simulink model "tank_warmup"  (R2024b)
settings: Solver=ode15s  StartTime=0.0  StopTime=100  RelTol=1e-3
undefined symbols (not defined in the file): AC_tank_weight, Ambient_temp
libraries: fl_lib x11, nesl_utility x7, SimscapeFluids_lib x3
settings Model: Creator=MW  LastModifiedBy=MW

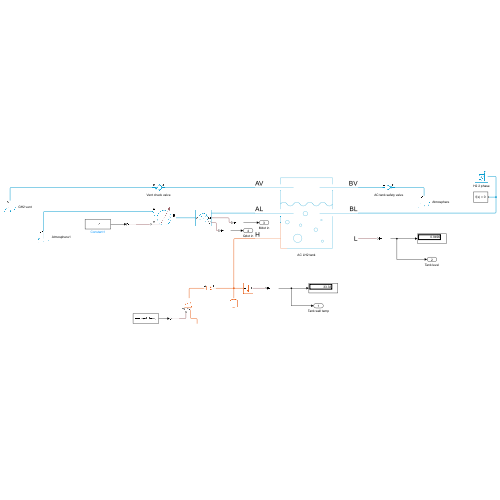
[thumbnail: Simulink's stored preview of the top-level diagram]
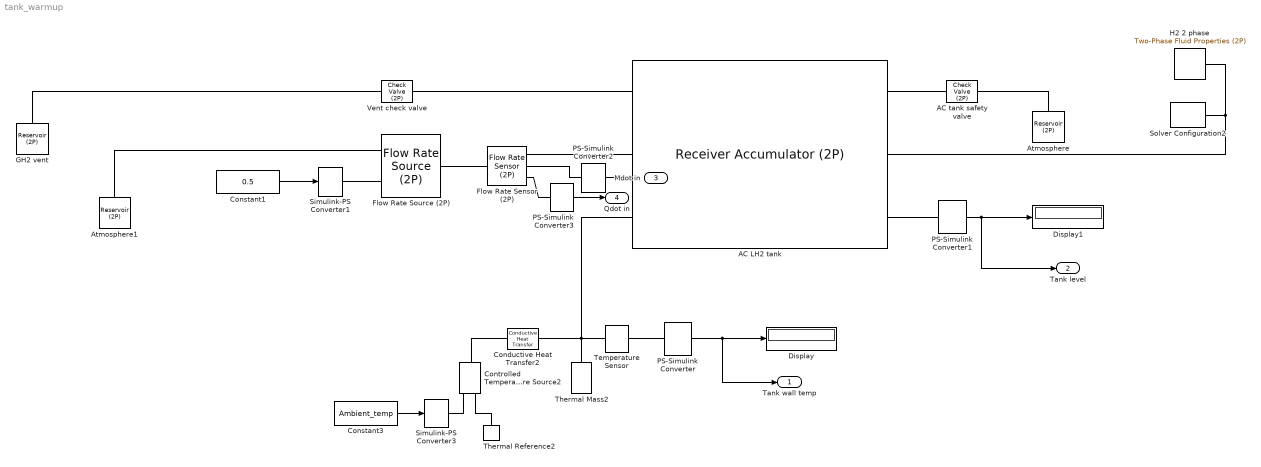
== system tank_warmup ==
  AC LH2 tank : SimscapeFluids_lib/Two-Phase Fluid/Tanks & Accumulators/Receiver Accumulator (2P)  volume=AC_tank_volume m^3  tank_area=AC_tank_cross_sectional_area m^2  area_AV=AC_return_line_port_inner_area m^2  area_BV=return_pipe_inner_area m^2  area_AL=AC_supply_line_port_inner_area m^2  area_BL=AC_engine_feed_port_inner_area m^2  V_frac_liq_error=simscape.enum.assert.action.none  V_frac_liq_min=0.05  V_frac_liq_max=0.95  V_frac_smooth=0.01  p_crit_error=simscape.enum.assert.action.error  hc_vap=AC_tank_vapour_heat_transfer_coeff W/(K*m^2)  hc_liq=AC_tank_liquid_heat_transfer_coeff W/(K*m^2)  p_init=3 bar  fraction_spec=fluids.two_phase_fluid.tanks_accumulators.enum.LiquidFractionSpec.Volume  M_frac_liq_init=0.5  V_frac_liq_init=0.9  saturated_init=false  energy_spec=fluids.two_phase_fluid.tanks_accumulators.enum.EnergySpec.Temperature  delta_T_sub_init=5 deltaK  delta_T_sup_init=5 deltaK  T_liq_init=20 K  T_vap_init=27 K  h_liq_init=400 kJ/kg  h_vap_init=2700 kJ/kg  u_liq_init=400 kJ/kg  u_vap_init=2700 kJ/kg  tau_vap_cond=0.1 s
      settings: InternalSimscapePortConfiguration="{\"Bottom\":[],\"Left\":[{\"id\":\"AV\",\"label\":\"AV\",\"type\":\"foundation.two_phase_fluid.two_phase_fluid\"},{\"id\":\"AL\",\"label\":\"AL\",\"type\":\"foundation.two_phase_fluid.two_phase_fluid\"},{\"id\":\"H\",\"label\":\"H\",\"type\":\"foundation.thermal.thermal\"}],\"Right\":[{\"id\":\"BV\",\"label\":\"BV\",\"type\":\"foundation.two_phase_fluid.two_phase_fluid\"},{\"id\":\"BL\",\"label\":\"BL\",\"type\":\"foundation.two_phase_fluid.two_phase_fluid\"},{\"id\":\"L\",\"label\":\"L\",\"type\":\"output\"}],\"Top\":[]}"
  AC tank safety valve : SimscapeFluids_lib/Two-Phase Fluid/Valves & Orifices/Directional Control Valves/Check Valve (2P)  liquid_valve_parameterization=fluids.two_phase_fluid.valves_orifices.enum.LiquidPressureValveParameterization.LinearArea  opening_pressure_spec=fluids.two_phase_fluid.valves_orifices.enum.PressureControlSpec.PressureDifferential  p_crack_differential=4.5 bar  p_crack_gauge=0.1 MPa  p_max_differential=4.9 bar  p_max_gauge=0.2 MPa  mdot_nominal_max=0.1 kg/s  delta_p_nominal_max=0.001 MPa  valve_area_max=AC_vent_valve_orifice_area m^2  p_diff_TLU=[0.2 : 0.2 : 1.2] MPa  p_gauge_TLU=[0.2 : 0.2 : 1.2] MPa  valve_area_TLU=[1e-10, 2e-06, 4e-06, 6e-06, 8e-06, 1e-05] m^2  energy_spec=foundation.enum.energy_spec.temperature  p_inlet=0.101325 MPa  T_inlet=293.15 K  x_inlet=0  alpha_inlet=0  h_inlet=400 kJ/kg  u_inlet=400 kJ/kg  Cd=AC_vent_valve_discharge_coeff  pressure_recovery=false  leakage_fraction=1e-9  smoothing_factor=0.01  B_lam=0.999  tau_x=0.1 s  area=AC_vent_line_port_inner_area m^2  vapor_valve_parameterization=fluids.two_phase_fluid.valves_orifices.enum.VaporOrificeParameterization.Cv  opening_characteristic=fluids.two_phase_fluid.valves_orifices.enum.OpeningCharacteristics.Linear  Cv_max=4  p_diff_Cv_TLU=0.2 : 0.2 : 1.2 MPa  p_gauge_Cv_TLU=0.2 : 0.2 : 1.2 MPa  Cv_TLU=[1e-06, .8, 1.6, 2.4, 3.2, 4]  xT_Cv=0.7  Kv_max=3.6  p_diff_Kv_TLU=0.2 : 0.2 : 1.2 MPa  p_gauge_Kv_TLU=0.2 : 0.2 : 1.2 MPa  Kv_TLU=[1e-06, .72, 1.44, 2.16, 2.88, 3.6]  xT_Kv=0.7  orifice_area_max=1e-4 m^2  p_diff_orifice_area_TLU=0.2 : 0.2 : 1.2 MPa  p_gauge_orifice_area_TLU=0.2 : 0.2 : 1.2 MPa  orifice_area_TLU=[1e-10, 2e-05, 4e-05, 6e-05, 8e-05, .0001] m^2
      settings: InternalSimscapePortConfiguration="{\"Bottom\":[],\"Left\":[{\"id\":\"A\",\"label\":\"A\",\"type\":\"foundation.two_phase_fluid.two_phase_fluid\"}],\"Right\":[{\"id\":\"B\",\"label\":\"B\",\"type\":\"foundation.two_phase_fluid.two_phase_fluid\"}],\"Top\":[]}"
  Atmosphere : fl_lib/Two-Phase Fluid/Elements/Reservoir (2P)  pressure_spec=foundation.enum.ReservoirPressureSpec2P.Specified  reservoir_pressure=0.101325 MPa  reservoir_condensing_temperature=373.15 K  reservoir_evaporating_temperature=373.15 K  energy_spec=foundation.enum.ReservoirEnergySpec2P.Temperature  reservoir_temperature=293.15 K  reservoir_quality=0.5  reservoir_void_fraction=0.5  reservoir_enthalpy=1500 kJ/kg  reservoir_internal_energy=1500 kJ/kg  reservoir_subcooling=5 deltaK  reservoir_superheating=5 deltaK  area_A=0.02 m^2
  Atmosphere1 : fl_lib/Two-Phase Fluid/Elements/Reservoir (2P)  pressure_spec=foundation.enum.ReservoirPressureSpec2P.Specified  reservoir_pressure=3.4 bar  reservoir_condensing_temperature=373.15 K  reservoir_evaporating_temperature=373.15 K  energy_spec=foundation.enum.ReservoirEnergySpec2P.Temperature  reservoir_temperature=293.15 K  reservoir_quality=0.5  reservoir_void_fraction=0.5  reservoir_enthalpy=1500 kJ/kg  reservoir_internal_energy=1500 kJ/kg  reservoir_subcooling=5 deltaK  reservoir_superheating=5 deltaK  area_A=AC_supply_line_port_inner_area m^2
  Conductive Heat Transfer2 : fl_lib/Thermal/Thermal Elements/Conductive Heat Transfer  thermal_type=foundation.enum.ConstantVariableTabulated.Constant  wall_geometry=foundation.enum.ConductionWallGeometry.Planar  area=AC_tank_surface_area m^2  thickness=AC_wall_thickness m  d_in=0.05 m  d_out=0.1 m  L=1 m  th_cond_min=10 W/(K*m)  th_cond=0.001 W/(m*K)  th_cond_TLU=[413, 401, 392, 383, 371, 357, 342] W/(K*m)  temp_TLU=[200, 273, 400, 600, 800, 1000, 1200] K  T_specify=off  T_priority=None  T=0 K  T_nominal_specify=off  T_nominal_value=1  T_nominal_unit=K  Q_specify=off  Q_priority=None  Q=0 W  Q_nominal_specify=off  Q_nominal_value=1  Q_nominal_unit=W
  Constant1 : Constant  Value=0.5
  Constant3 : Constant  Value=Ambient_temp
  Controlled Temperature Source2 : fl_lib/Thermal/Thermal Sources/Controlled Temperature Source
  Display : Display
  Display1 : Display
  Flow Rate Sensor (2P) : fl_lib/Two-Phase Fluid/Sensors/Flow Rate Sensor (2P)  mass_flow_measure=true  volumetric_flow_measure=true  energy_flow_measure=false
      settings: InternalSimscapePortConfiguration="{\"Bottom\":[],\"Left\":[{\"id\":\"A\",\"label\":\"A\",\"type\":\"foundation.two_phase_fluid.two_phase_fluid\"}],\"Right\":[{\"id\":\"B\",\"label\":\"B\",\"type\":\"foundation.two_phase_fluid.two_phase_fluid\"},{\"id\":\"M\",\"label\":\"M\",\"type\":\"output\"},{\"id\":\"V\",\"label\":\"V\",\"type\":\"output\"}],\"Top\":[]}"
  Flow Rate Source (2P) : fl_lib/Two-Phase Fluid/Sources/Flow Rate Source (2P)  source_type=foundation.enum.constant_controlled.controlled  flow_type=foundation.enum.mass_volumetric_flow.volumetric  mass_flow=0 kg/s  volumetric_flow=0 m^3/s  power_spec=foundation.enum.power_spec.isentropic  area_A=AC_supply_line_port_inner_area m^2  area_B=AC_supply_line_port_inner_area m^2
      settings: InternalSimscapePortConfiguration="{\"Bottom\":[],\"Left\":[{\"id\":\"A\",\"label\":\"A\",\"type\":\"foundation.two_phase_fluid.two_phase_fluid\"},{\"id\":\"V\",\"label\":\"V\",\"type\":\"input\"}],\"Right\":[{\"id\":\"B\",\"label\":\"B\",\"type\":\"foundation.two_phase_fluid.two_phase_fluid\"}],\"Top\":[]}"
  GH2 vent : fl_lib/Two-Phase Fluid/Elements/Reservoir (2P)  pressure_spec=foundation.enum.ReservoirPressureSpec2P.Specified  reservoir_pressure=3 bar  reservoir_condensing_temperature=373.15 K  reservoir_evaporating_temperature=373.15 K  energy_spec=foundation.enum.ReservoirEnergySpec2P.Temperature  reservoir_temperature=293.15 K  reservoir_quality=0.5  reservoir_void_fraction=0.5  reservoir_enthalpy=1500 kJ/kg  reservoir_internal_energy=1500 kJ/kg  reservoir_subcooling=5 deltaK  reservoir_superheating=5 deltaK  area_A=AC_supply_line_port_inner_area m^2
  H2 2 phase : fl_lib/Two-Phase Fluid/Utilities/Two-Phase Fluid Properties (2P)  u_min=H2Tables.u_min kJ/kg  u_max=H2Tables.u_max kJ/kg  p_TLU=H2Tables.p MPa  p_crit=H2Tables.p_crit MPa  critical_region=foundation.enum.critical_region.clip  p_crit_fraction=0.12  p_atm=0.101325 MPa  properties_range_check=simscape.enum.assert.action.error  q_rev=0.01 Pa  unorm_liq=H2Tables.liquid.unorm  v_liq=H2Tables.liquid.v m^3/kg  s_liq=H2Tables.liquid.s kJ/(kg*K)  T_liq=H2Tables.liquid.T K  nu_liq=H2Tables.liquid.nu mm^2/s  k_liq=H2Tables.liquid.k W/(m*K)  Pr_liq=H2Tables.liquid.Pr  u_sat_liq=H2Tables.liquid.u_sat kJ/kg  unorm_vap=H2Tables.vapor.unorm  v_vap=H2Tables.vapor.v m^3/kg  s_vap=H2Tables.vapor.s kJ/(kg*K)  T_vap=H2Tables.vapor.T K  nu_vap=H2Tables.vapor.nu mm^2/s  k_vap=H2Tables.vapor.k W/(m*K)  Pr_vap=H2Tables.vapor.Pr  u_sat_vap=H2Tables.vapor.u_sat kJ/kg
      settings: InternalSimscapePortConfiguration="{\"Bottom\":[],\"Left\":[],\"Right\":[{\"id\":\"A\",\"label\":\"\",\"type\":\"foundation.two_phase_fluid.two_phase_fluid\"}],\"Top\":[]}"
  PS-Simulink Converter{,1..3} (4 alike) : nesl_utility/PS-Simulink Converter  PhysicalDomain=network_engine_domain  SubClassName=ps_output  LeftPortType=input  RightPortType=output  PseudoPeriodic=off  Frequencies=[]  VectorFormat=inherit  Unit=inherit  AffineConversion=off
  Simulink-PS Converter1 : nesl_utility/Simulink-PS Converter  PhysicalDomain=network_engine_domain  SubClassName=ps_input  LeftPortType=input  RightPortType=output  PseudoPeriodic=off  Frequencies=[]  NoiseDistribution=none  NoiseParameters=[]  Unit=1  AffineConversion=off  FilteringAndDerivatives=zero  SimscapeFilterOrder=1  InputFilterTimeConstant=0.001  UdotUserProvided=1
  Simulink-PS Converter3 : nesl_utility/Simulink-PS Converter  PhysicalDomain=network_engine_domain  SubClassName=ps_input  LeftPortType=input  RightPortType=output  PseudoPeriodic=off  Frequencies=[]  NoiseDistribution=none  NoiseParameters=[]  Unit=1  AffineConversion=off  FilteringAndDerivatives=zero  SimscapeFilterOrder=1  InputFilterTimeConstant=0.001  UdotUserProvided=1
  Solver Configuration2 : nesl_utility/Solver Configuration  PhysicalDomain=network_engine_domain  SubClassName=solver  LeftPortType=input  RightPortType=generic  Tones=[]  Harmonics=[]  SimulateNoise=off  Profile=off  UseLocalSampling=off  EnableSwitchedLinearOptims=on  FrequencyDomain=off  UseCCode=off  RelTol=0.001  AbsTol=0.001  MinStep=1e-09  ToWorkspace=off  RevertToSquareIcSolve=off  NumHomotopyIterations=100  PhasorMode=off  PhasorModeNumHarmonics=1  ConsistencySolver=NEWTON_XTOL_AFTER_FTOL  IndexReductionMethod=DerivativeReplacement  DoDC=off  ResidualTolerance=1e-09  ConsistencyTolSource=GLOBAL  ConsistencyAbsTol=0.001  ConsistencyRelTol=0.001  ConsistencyTolFactor=1e-7  UseLocalSolver=off  LocalSolverChoice=NE_TRAPEZOIDAL_ADVANCER  ResolveIndetEquations=on  FunctionEvalNumThread=1  LocalSolverSampleTime=1e-3  DoFixedCost=off  MaxNonlinIter=3  MaxModeIter=2  ComputeImpulses=off  ImpulseIterations=2  LinearAlgebra=auto  LinearAlgebraNumThread=0  EquationFormulation=NE_TIME_EF  DelaysMemoryBudget=1024  AutomaticFiltering=on  FilteringTimeConstant=0.001  PartitionStorageMethod=AS_NEEDED  PartitionMemoryBudget=1024  PartitionMethod=ROBUST  MultibodyUseLocalSolver=off  MultibodyLocalSolverChoice=ODE1  MultibodyLocalSolverSampleTime=0.001
  Temperature Sensor : fl_lib/Thermal/Thermal Sensors/Temperature Sensor  temperature_measure=foundation.enum.MeasurementReference.absolute
      settings: InternalSimscapePortConfiguration="{\"Bottom\":[],\"Left\":[{\"id\":\"A\",\"label\":\"A\",\"type\":\"foundation.thermal.thermal\"}],\"Right\":[{\"id\":\"T\",\"label\":\"T\",\"type\":\"output\"}],\"Top\":[]}"
  Thermal Mass2 : fl_lib/Thermal/Thermal Elements/Thermal Mass  mass_type=foundation.enum.constant_variable.constant  mass=AC_tank_weight/2 kg  sp_heat=250 J/kg/K  mass_min=1e-6 kg  num_ports=foundation.enum.numPorts2.one  m_specify=off  m_priority=High  m=1 kg  m_nominal_specify=off  m_nominal_value=1  m_nominal_unit=kg  T_specify=on  T_priority=High  T=20 K  T_nominal_specify=off  T_nominal_value=1  T_nominal_unit=K  Q_specify=off  Q_priority=None  Q=0 W  Q_nominal_specify=off  Q_nominal_value=1  Q_nominal_unit=W
  Thermal Reference2 : fl_lib/Thermal/Thermal Elements/Thermal Reference
  Vent check valve : SimscapeFluids_lib/Two-Phase Fluid/Valves & Orifices/Directional Control Valves/Check Valve (2P)  liquid_valve_parameterization=fluids.two_phase_fluid.valves_orifices.enum.LiquidPressureValveParameterization.LinearArea  opening_pressure_spec=fluids.two_phase_fluid.valves_orifices.enum.PressureControlSpec.PressureDifferential  p_crack_differential=2.5 bar  p_crack_gauge=0.1 MPa  p_max_differential=3 bar  p_max_gauge=0.2 MPa  mdot_nominal_max=0.1 kg/s  delta_p_nominal_max=0.001 MPa  valve_area_max=return_valve_orifice_area m^2  p_diff_TLU=[0.2 : 0.2 : 1.2] MPa  p_gauge_TLU=[0.2 : 0.2 : 1.2] MPa  valve_area_TLU=[1e-10, 2e-06, 4e-06, 6e-06, 8e-06, 1e-05] m^2  energy_spec=foundation.enum.energy_spec.temperature  p_inlet=0.101325 MPa  T_inlet=293.15 K  x_inlet=0  alpha_inlet=0  h_inlet=400 kJ/kg  u_inlet=400 kJ/kg  Cd=GS_vent_discharge_coeff  pressure_recovery=false  leakage_fraction=1e-9  smoothing_factor=0.01  B_lam=valve_laminar_p_ratio  tau_x=0.1 s  area=return_pipe_inner_area m^2  vapor_valve_parameterization=fluids.two_phase_fluid.valves_orifices.enum.VaporOrificeParameterization.Cv  opening_characteristic=fluids.two_phase_fluid.valves_orifices.enum.OpeningCharacteristics.Linear  Cv_max=4  p_diff_Cv_TLU=0.2 : 0.2 : 1.2 MPa  p_gauge_Cv_TLU=0.2 : 0.2 : 1.2 MPa  Cv_TLU=[1e-06, .8, 1.6, 2.4, 3.2, 4]  xT_Cv=0.7  Kv_max=3.6  p_diff_Kv_TLU=0.2 : 0.2 : 1.2 MPa  p_gauge_Kv_TLU=0.2 : 0.2 : 1.2 MPa  Kv_TLU=[1e-06, .72, 1.44, 2.16, 2.88, 3.6]  xT_Kv=0.7  orifice_area_max=1e-4 m^2  p_diff_orifice_area_TLU=0.2 : 0.2 : 1.2 MPa  p_gauge_orifice_area_TLU=0.2 : 0.2 : 1.2 MPa  orifice_area_TLU=[1e-10, 2e-05, 4e-05, 6e-05, 8e-05, .0001] m^2
      settings: InternalSimscapePortConfiguration="{\"Bottom\":[],\"Left\":[{\"id\":\"A\",\"label\":\"A\",\"type\":\"foundation.two_phase_fluid.two_phase_fluid\"}],\"Right\":[{\"id\":\"B\",\"label\":\"B\",\"type\":\"foundation.two_phase_fluid.two_phase_fluid\"}],\"Top\":[]}"
  Tank wall temp : Outport
  Tank level : Outport  Port=2
  Mdot in : Outport  Port=3
  Qdot in : Outport  Port=4
  wires:
  Constant3/1 -> Simulink-PS Converter3/1
  PS-Simulink Converter/1 -> Display/1, Tank wall temp/1
  PS-Simulink Converter1/1 -> Tank level/1, Display1/1
  Constant1/1 -> Simulink-PS Converter1/1
  PS-Simulink Converter2/1 -> Mdot in/1
  PS-Simulink Converter3/1 -> Qdot in/1
  connections:
  Conductive Heat Transfer2/RConn1 -- AC LH2 tank/LConn3 -- Thermal Mass2/LConn1 -- Temperature Sensor/LConn1
  PS-Simulink Converter/LConn1 -- Temperature Sensor/RConn1
  Simulink-PS Converter3/RConn1 -- Controlled Temperature Source2/RConn1
  PS-Simulink Converter1/LConn1 -- AC LH2 tank/RConn3
  Thermal Reference2/LConn1 -- Controlled Temperature Source2/RConn2
  Vent check valve/LConn1 -- AC LH2 tank/LConn1
  Atmosphere1/LConn1 -- Flow Rate Source (2P)/LConn1
  Conductive Heat Transfer2/LConn1 -- Controlled Temperature Source2/LConn1
  AC LH2 tank/RConn1 -- AC tank safety valve/LConn1
  AC LH2 tank/RConn2 -- H2 2 phase/RConn1 -- Solver Configuration2/RConn1
  AC tank safety valve/RConn1 -- Atmosphere/LConn1
  GH2 vent/LConn1 -- Vent check valve/RConn1
  Simulink-PS Converter1/RConn1 -- Flow Rate Source (2P)/LConn2
  Flow Rate Source (2P)/RConn1 -- Flow Rate Sensor (2P)/LConn1
  Flow Rate Sensor (2P)/RConn1 -- AC LH2 tank/LConn2
  Flow Rate Sensor (2P)/RConn2 -- PS-Simulink Converter2/LConn1
  PS-Simulink Converter3/LConn1 -- Flow Rate Sensor (2P)/RConn3
